simulink model "anaht"  (R2018a)
settings: Solver=VariableStepAuto  StartTime=0.0  StopTime=1.0  RelTol=1e-3
libraries: powerlib x20
settings Model: Creator=hp  LastModifiedBy=hp

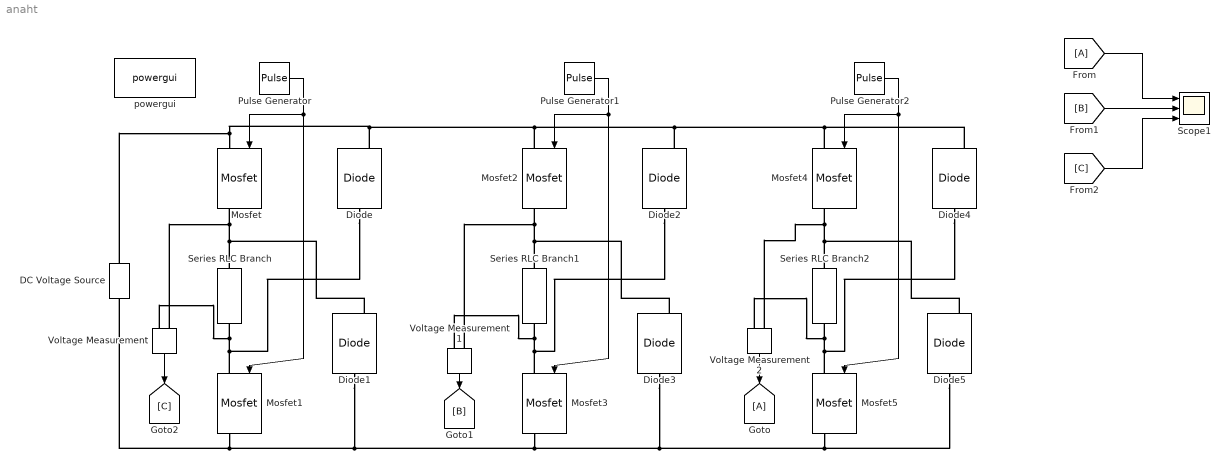
== system anaht ==
  DC Voltage Source : powerlib/Electrical Sources/DC Voltage Source  Amplitude=24  Measurements=None
  Diode{,1..5} (6 alike) : powerlib/Power Electronics/Diode  Ron=0.001  Lon=0  Vf=0.8  IC=0  UseSnubber=0  Rs=500  Cs=250e-9  Measurements=on
  Mosfet{,1..5} (6 alike) : powerlib/Power Electronics/Mosfet  Ron=0.1  Lon=0  Rd=0.01  Vfd=0  IC=0  Rs=1e5  Cs=inf  Measurements=on
  Pulse Generator : DiscretePulseGenerator  PulseType=Time based  Period=5e-01  PulseWidth=120*100/360  PhaseDelay=5e-01*2/3
  Pulse Generator1 : DiscretePulseGenerator  PulseType=Time based  Period=5e-01  PulseWidth=120*100/360  PhaseDelay=5e-01/3
  Pulse Generator2 : DiscretePulseGenerator  PulseType=Time based  Period=5e-01  PulseWidth=120*100/360
  Scope1 : Scope  NumInputPorts=3
  Series RLC Branch : powerlib/Elements/Series RLC Branch  LConnTagsString=__new0  RConnTagsString=__new0  BranchType=R  Resistance=1  Inductance=1  SetiL0=off  InitialCurrent=0  Capacitance=1e-6  Setx0=off  InitialVoltage=0  Measurements=None
  Series RLC Branch1 : powerlib/Elements/Series RLC Branch  LConnTagsString=__new0  RConnTagsString=__new0  BranchType=R  Resistance=1  Inductance=1  SetiL0=off  InitialCurrent=0  Capacitance=1e-6  Setx0=off  InitialVoltage=0  Measurements=None
  Series RLC Branch2 : powerlib/Elements/Series RLC Branch  LConnTagsString=__new0  RConnTagsString=__new0  BranchType=R  Resistance=1  Inductance=1  SetiL0=off  InitialCurrent=0  Capacitance=1e-6  Setx0=off  InitialVoltage=0  Measurements=None
  Voltage Measurement : powerlib/Measurements/Voltage Measurement  PhasorSimulation=off  OutputType=Complex  PSBequivalent=0
  Voltage Measurement1 : powerlib/Measurements/Voltage Measurement  PhasorSimulation=off  OutputType=Complex  PSBequivalent=0
  Voltage Measurement2 : powerlib/Measurements/Voltage Measurement  PhasorSimulation=off  OutputType=Complex  PSBequivalent=0
  powergui : powerlib/powergui  Priority=1  SimulationMode=Discrete  SampleTime=5e-6  frequency=60  Iterations=50  frequencyindice=0  Pbase=100e6  ErrMax=1e-4  UnitsV=kV  UnitsW=MW  buscounter=0  FunctionMessages=off  echomessages=off  EnableUseOfTLC=off  CurrentSourceSwitches=off  DisableSnubberDevices=off  DisableRonSwitches=off  DisableVfSwitches=off  DisplayEquations=off  SolverType=Tustin/Backward Euler (TBE)  Interpol=off  ExternalGateDelay=off  methode=off  Ts=100  x0status=blocks  SPID=on  SwTol=0  HookPort=off  RestoreLinks=warning  ResistiveCurrentMeasurement=off  Frange=[0:2:500]  Ylog=off  Xlog=on  ShowGrid=off  save=off  variable=ZData  structure=0  ZoomFFT=off  StartTime=0.0  cycles=1  DisplayStyle=1  fundamental=60  FreqAxis=off  MaxFrequency=1000  frequencyindicesteady=1  RmsSteady=1  display=off
  wires:
  Pulse Generator/1 -> Mosfet1/1, Mosfet/1
  Pulse Generator2/1 -> Mosfet5/1, Mosfet4/1
  Pulse Generator1/1 -> Mosfet3/1, Mosfet2/1
  Voltage Measurement2/1 -> [A]
  Voltage Measurement1/1 -> [B]
  [C] -> Scope1/3
  [B] -> Scope1/2
  [A] -> Scope1/1
  Voltage Measurement/1 -> [C]
  connections:
  Series RLC Branch2/LConn1 -- Diode5/RConn1 -- Voltage Measurement2/LConn1 -- Mosfet4/RConn1
  Voltage Measurement2/LConn2 -- Diode4/LConn1 -- Mosfet5/LConn1 -- Series RLC Branch2/RConn1
  Diode5/LConn1 -- Mosfet3/RConn1 -- DC Voltage Source/LConn1 -- Mosfet1/RConn1 -- Diode1/LConn1 -- Diode3/LConn1 -- Mosfet5/RConn1
  Diode/RConn1 -- DC Voltage Source/RConn1 -- Mosfet/LConn1 -- Mosfet4/LConn1 -- Diode4/RConn1 -- Diode2/RConn1 -- Mosfet2/LConn1
  Voltage Measurement1/LConn2 -- Series RLC Branch1/RConn1 -- Diode2/LConn1 -- Mosfet3/LConn1
  Mosfet2/RConn1 -- Voltage Measurement1/LConn1 -- Diode3/RConn1 -- Series RLC Branch1/LConn1
  Voltage Measurement/LConn2 -- Diode/LConn1 -- Mosfet1/LConn1 -- Series RLC Branch/RConn1
  Series RLC Branch/LConn1 -- Diode1/RConn1 -- Voltage Measurement/LConn1 -- Mosfet/RConn1
